simulink model "Strt_DD"  (R2016b)
settings: configuration reference "CodeGenConfigSet" (kept outside this file)
values from neighbouring files (symbols this model uses):
  Strt_stPsDiaDisbl_C = Calibration.Parameter    [init_Strt_DD.m]    (also in init_Strt_DD_SIL.m = Simulink.Parameter)
  Strt_stPsDisbl_C = Calibration.Parameter    [init_Strt_DD.m]    (also in init_Strt_DD_SIL.m = Simulink.Parameter)
libraries: simulink x1
settings Model: Creator=xuxingpei  LastModifiedBy=xuxingpei
settings ConfigSetRef: SourceLocation=Base Workspace

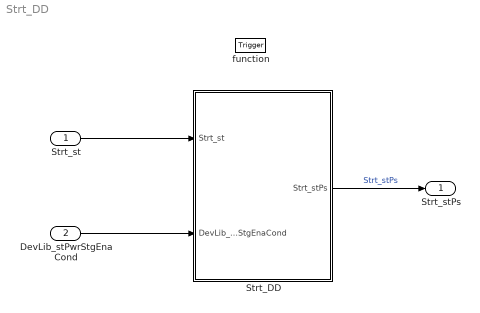
== system Strt_DD ==
  Strt_st : Inport  Description=Control signal for the starter relay  OutMin=0  OutMax=1  OutDataTypeStr=boolean
  DevLib_stPwrStgEnaCond : Inport  Description=Control unit status relevant to power stage deactivation/error diagnosis  Port=2  OutMin=0  OutMax=65535  OutDataTypeStr=State_uint16
  function : TriggerPort  TriggerType=function-call  VariantControl=Variant
  Strt_DD : Subsystem
  Strt_stPs : Outport  Description=Status of starter power stage  OutMin=0  OutMax=1  OutDataTypeStr=boolean
  wires:
  Strt_st/1 -> Strt_DD/1(Strt_st)
  DevLib_stPwrStgEnaCond/1 -> Strt_DD/2(DevLib_stPwrStgEnaCond)
  Strt_DD/1(Strt_stPs) -> Strt_stPs/1  "Strt_stPs"

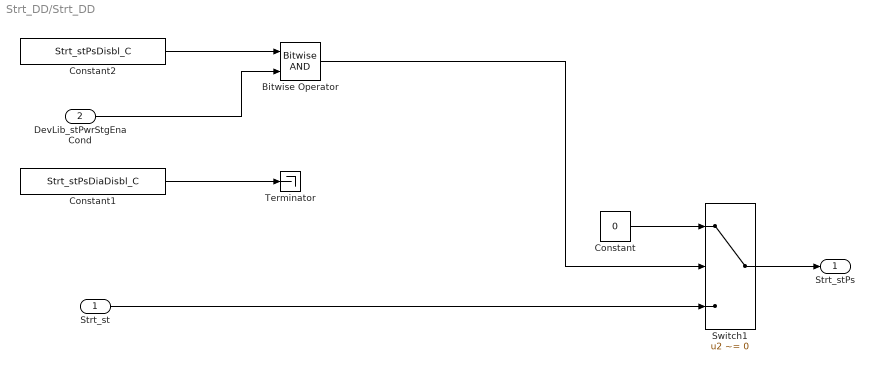
== system Strt_DD/Strt_DD ==
  Strt_st : Inport  Description=Control signal for the starter relay  OutMin=0  OutMax=1  OutDataTypeStr=boolean
  DevLib_stPwrStgEnaCond : Inport  Description=Control unit status relevant to power stage deactivation/error diagnosis  Port=2  OutMin=0  OutMax=65535  OutDataTypeStr=State_uint16
  Bitwise Operator : simulink/Logic and Bit Operations/Bitwise Operator  logicop=AND  UseBitMask=off  NumInputPorts=2  BitMask=bin2dec('11011001')  BitMaskRealWorld=Stored Integer
  Constant : Constant  Value=0  OutDataTypeStr=Inherit: Inherit via back propagation
  Constant1 : Constant  Value=Strt_stPsDiaDisbl_C
  Constant2 : Constant  Value=Strt_stPsDisbl_C
  Switch1 : Switch  Criteria=u2 ~= 0  InputSameDT=on
  Terminator : Terminator
  Strt_stPs : Outport  Description=Status of starter power stage  OutMin=0  OutMax=1  OutDataTypeStr=boolean
  wires:
  Constant2/1 -> Bitwise Operator/1
  DevLib_stPwrStgEnaCond/1 -> Bitwise Operator/2
  Constant1/1 -> Terminator/1
  Bitwise Operator/1 -> Switch1/2
  Switch1/1 -> Strt_stPs/1
  Strt_st/1 -> Switch1/3
  Constant/1 -> Switch1/1
